simulink model "AMR_main_23b"  (R2024a)
settings: configuration reference "Configuration" (kept outside this file)
model workspace (MAT data in the model file):
  RTK_health_condition = 30
  mdlWSDbList : string (value not decoded)
undefined symbols (not defined in the file or in its folder): Down, Pull
libraries: speedgoatlib_IO60X_IO69X x17, tramontina_database_nvidialib x11, tramontina_database_curtislib x7, tramontina_database_xsenslib x4, tramontina_database_moboticlib x4, speedgoatlib_IO691 x3, canmsglib x2, slrealtimeseriallib x2, etargetslib x1, tramontina_database_sick_modbuslib x1
(part 2 of 2)

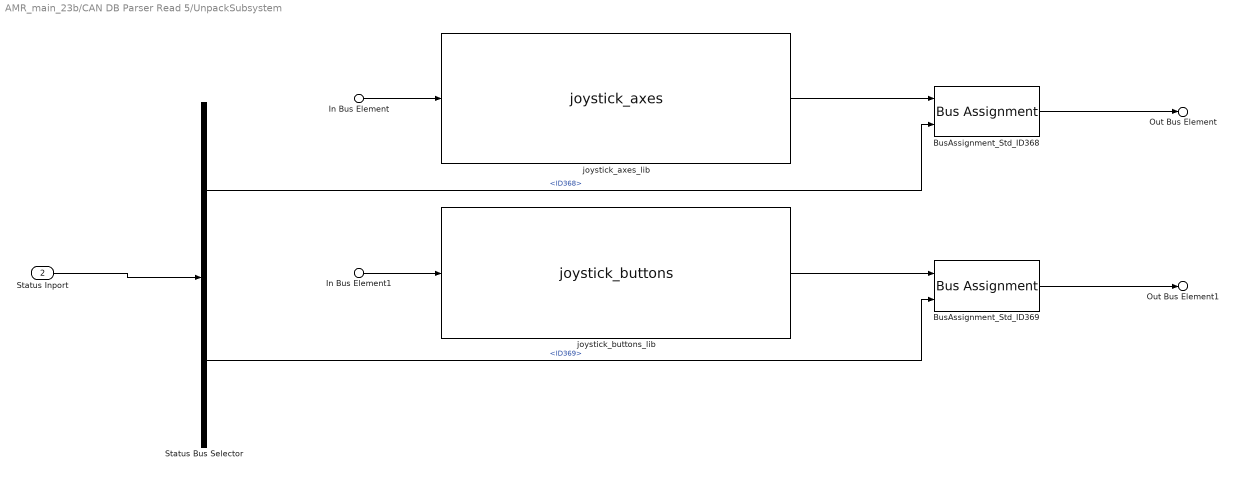
== system AMR_main_23b/CAN DB Parser Read 5/UnpackSubsystem ==
  In Bus Element : Inport  PortName=Unpack_In  Element=Std.ID368
  In Bus Element1 : Inport  PortName=Unpack_In  Element=Std.ID369
  Status Inport : Inport  Port=2
  BusAssignment_Std_ID368 : BusAssignment  AssignedSignals=MessageStatus.Status
  BusAssignment_Std_ID369 : BusAssignment  AssignedSignals=MessageStatus.Status
  Status Bus Selector : BusSelector  OutputSignals=Std.ID368,Std.ID369
  joystick_axes_lib : tramontina_database_nvidialib/CAN unpack/joystick_axes  SystemSampleTime=-1  VariantActivationTime=update diagram  AllowFlexibleInterface=on  Latency=0  AutoFrameSizeCalculation=off
  joystick_buttons_lib : tramontina_database_nvidialib/CAN unpack/joystick_buttons  SystemSampleTime=-1  VariantActivationTime=update diagram  AllowFlexibleInterface=on  Latency=0  AutoFrameSizeCalculation=off
  Out Bus Element : Outport  PortName=Unpack_Out  Element=ID368_joystick_axes
  Out Bus Element1 : Outport  PortName=Unpack_Out  Element=ID369_joystick_buttons
  wires:
  In Bus Element/1 -> joystick_axes_lib/1
  joystick_axes_lib/1 -> BusAssignment_Std_ID368/1
  BusAssignment_Std_ID368/1 -> Out Bus Element/1
  In Bus Element1/1 -> joystick_buttons_lib/1
  joystick_buttons_lib/1 -> BusAssignment_Std_ID369/1
  BusAssignment_Std_ID369/1 -> Out Bus Element1/1
  Status Inport/1 -> Status Bus Selector/1
  Status Bus Selector/1 -> BusAssignment_Std_ID368/2  "<ID368>"
  Status Bus Selector/2 -> BusAssignment_Std_ID369/2  "<ID369>"

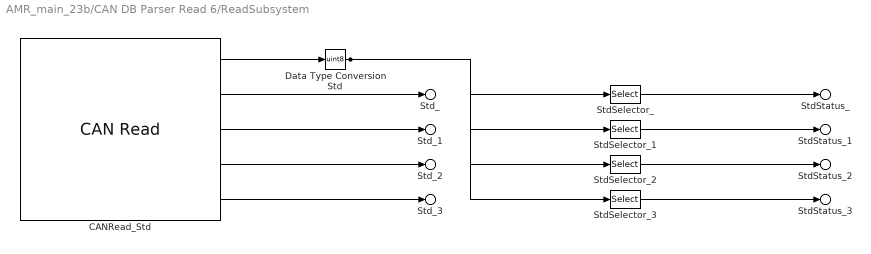
== system AMR_main_23b/CAN DB Parser Read 6/ReadSubsystem ==
  CANRead_Std : speedgoatlib_IO60X_IO69X/CAN/CAN Read   moduleType=IO691  id=1  channel=1  canType=CAN (HS)  messageType=CAN (HS)  useBusOut=on  HasMulRead=Specify by IDs  MsgIDlist="[370  371  372  373]"  isEFF=off  LabelInHex=off  enableInput=off  initValues=[691 1 0.005 0 1 1 0 1 2 0 4 370 371 372 373]  ts=5e-3
  Data Type ConversionStd : DataTypeConversion  OutDataTypeStr=uint8  SaturateOnIntegerOverflow=off  RndMeth=Floor
  StdSelector_ : Selector  IndexOptions=Index vector (dialog)  Indices=1  OutputSizes=1
  StdSelector_1 : Selector  IndexOptions=Index vector (dialog)  Indices=2  OutputSizes=1
  StdSelector_2 : Selector  IndexOptions=Index vector (dialog)  Indices=3  OutputSizes=1
  StdSelector_3 : Selector  IndexOptions=Index vector (dialog)  Indices=4  OutputSizes=1
  Std_ : Outport  PortName=Raw_Rx  Element=Std.ID370
  Std_1 : Outport  PortName=Raw_Rx  Element=Std.ID371
  Std_2 : Outport  PortName=Raw_Rx  Element=Std.ID372
  Std_3 : Outport  PortName=Raw_Rx  Element=Std.ID373
  StdStatus_ : Outport  Port=2  PortName=Status_Rx  Element=Std.ID370
  StdStatus_1 : Outport  Port=2  PortName=Status_Rx  Element=Std.ID371
  StdStatus_2 : Outport  Port=2  PortName=Status_Rx  Element=Std.ID372
  StdStatus_3 : Outport  Port=2  PortName=Status_Rx  Element=Std.ID373
  wires:
  CANRead_Std/1 -> Data Type ConversionStd/1
  CANRead_Std/2 -> Std_/1
  CANRead_Std/3 -> Std_1/1
  CANRead_Std/4 -> Std_2/1
  CANRead_Std/5 -> Std_3/1
  Data Type ConversionStd/1 -> StdSelector_/1, StdSelector_1/1, StdSelector_2/1, StdSelector_3/1
  StdSelector_/1 -> StdStatus_/1
  StdSelector_1/1 -> StdStatus_1/1
  StdSelector_2/1 -> StdStatus_2/1
  StdSelector_3/1 -> StdStatus_3/1

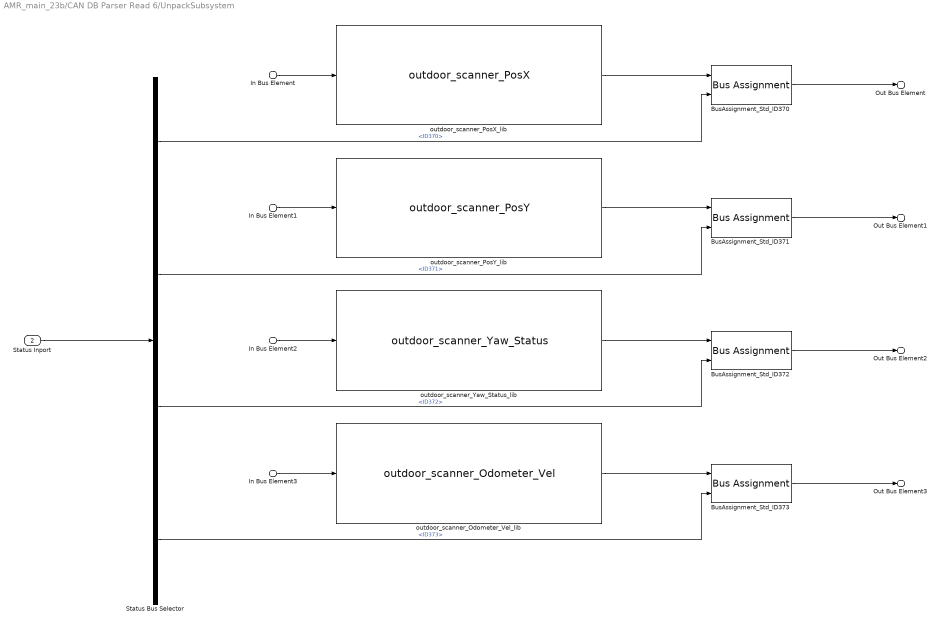
== system AMR_main_23b/CAN DB Parser Read 6/UnpackSubsystem ==
  In Bus Element : Inport  PortName=Unpack_In  Element=Std.ID370
  In Bus Element1 : Inport  PortName=Unpack_In  Element=Std.ID371
  In Bus Element2 : Inport  PortName=Unpack_In  Element=Std.ID372
  In Bus Element3 : Inport  PortName=Unpack_In  Element=Std.ID373
  Status Inport : Inport  Port=2
  BusAssignment_Std_ID{370..373} (4 alike) : BusAssignment  AssignedSignals=MessageStatus.Status
  Status Bus Selector : BusSelector  OutputSignals=Std.ID370,Std.ID371,Std.ID372,Std.ID373
  outdoor_scanner_Odometer_Vel_lib : tramontina_database_nvidialib/CAN unpack/outdoor_scanner_Odometer_Vel  SystemSampleTime=-1  VariantActivationTime=update diagram  AllowFlexibleInterface=on  Latency=0  AutoFrameSizeCalculation=off
  outdoor_scanner_PosX_lib : tramontina_database_nvidialib/CAN unpack/outdoor_scanner_PosX  SystemSampleTime=-1  VariantActivationTime=update diagram  AllowFlexibleInterface=on  Latency=0  AutoFrameSizeCalculation=off
  outdoor_scanner_PosY_lib : tramontina_database_nvidialib/CAN unpack/outdoor_scanner_PosY  SystemSampleTime=-1  VariantActivationTime=update diagram  AllowFlexibleInterface=on  Latency=0  AutoFrameSizeCalculation=off
  outdoor_scanner_Yaw_Status_lib : tramontina_database_nvidialib/CAN unpack/outdoor_scanner_Yaw_Status  SystemSampleTime=-1  VariantActivationTime=update diagram  AllowFlexibleInterface=on  Latency=0  AutoFrameSizeCalculation=off
  Out Bus Element : Outport  PortName=Unpack_Out  Element=ID370_outdoor_scanner_PosX
  Out Bus Element1 : Outport  PortName=Unpack_Out  Element=ID371_outdoor_scanner_PosY
  Out Bus Element2 : Outport  PortName=Unpack_Out  Element=ID372_outdoor_scanner_Yaw_Status
  Out Bus Element3 : Outport  PortName=Unpack_Out  Element=ID373_outdoor_scanner_Odometer_Vel
  wires:
  In Bus Element/1 -> outdoor_scanner_PosX_lib/1
  outdoor_scanner_PosX_lib/1 -> BusAssignment_Std_ID370/1
  BusAssignment_Std_ID370/1 -> Out Bus Element/1
  In Bus Element1/1 -> outdoor_scanner_PosY_lib/1
  outdoor_scanner_PosY_lib/1 -> BusAssignment_Std_ID371/1
  BusAssignment_Std_ID371/1 -> Out Bus Element1/1
  In Bus Element2/1 -> outdoor_scanner_Yaw_Status_lib/1
  outdoor_scanner_Yaw_Status_lib/1 -> BusAssignment_Std_ID372/1
  BusAssignment_Std_ID372/1 -> Out Bus Element2/1
  In Bus Element3/1 -> outdoor_scanner_Odometer_Vel_lib/1
  outdoor_scanner_Odometer_Vel_lib/1 -> BusAssignment_Std_ID373/1
  BusAssignment_Std_ID373/1 -> Out Bus Element3/1
  Status Inport/1 -> Status Bus Selector/1
  Status Bus Selector/1 -> BusAssignment_Std_ID370/2  "<ID370>"
  Status Bus Selector/2 -> BusAssignment_Std_ID371/2  "<ID371>"
  Status Bus Selector/3 -> BusAssignment_Std_ID372/2  "<ID372>"
  Status Bus Selector/4 -> BusAssignment_Std_ID373/2  "<ID373>"

== system AMR_main_23b/CAN DB Parser Read 7/ReadSubsystem ==
  CANRead_Std : speedgoatlib_IO60X_IO69X/CAN/CAN Read   moduleType=IO691  id=1  channel=1  canType=CAN (HS)  messageType=CAN (HS)  useBusOut=on  HasMulRead=Specify by IDs  MsgIDlist=[1459]  isEFF=off  LabelInHex=off  enableInput=off  initValues=[691 1 0.005 0 1 1 0 1 2 0 1 1459]  ts=5e-3
  Data Type ConversionStd : DataTypeConversion  OutDataTypeStr=uint8  SaturateOnIntegerOverflow=off  RndMeth=Floor
  StdSelector_ : Selector  IndexOptions=Index vector (dialog)  Indices=1  OutputSizes=1
  Std_ : Outport  PortName=Raw_Rx  Element=Std.ID1459
  StdStatus_ : Outport  Port=2  PortName=Status_Rx  Element=Std.ID1459
  wires:
  CANRead_Std/1 -> Data Type ConversionStd/1
  CANRead_Std/2 -> Std_/1
  Data Type ConversionStd/1 -> StdSelector_/1
  StdSelector_/1 -> StdStatus_/1

== system AMR_main_23b/CAN DB Parser Read 7/UnpackSubsystem ==
  In Bus Element : Inport  PortName=Unpack_In  Element=Std.ID1459
  Status Inport : Inport  Port=2
  BusAssignment_Std_ID1459 : BusAssignment  AssignedSignals=MessageStatus.Status
  Status Bus Selector : BusSelector  OutputSignals=Std.ID1459
  feedback_word_lib : tramontina_database_moboticlib/CAN unpack/feedback_word  SystemSampleTime=-1  VariantActivationTime=update diagram  AllowFlexibleInterface=on  Latency=0  AutoFrameSizeCalculation=off
  Out Bus Element : Outport  PortName=Unpack_Out  Element=ID1459_feedback_word
  wires:
  In Bus Element/1 -> feedback_word_lib/1
  feedback_word_lib/1 -> BusAssignment_Std_ID1459/1
  BusAssignment_Std_ID1459/1 -> Out Bus Element/1
  Status Inport/1 -> Status Bus Selector/1
  Status Bus Selector/1 -> BusAssignment_Std_ID1459/2  "<ID1459>"

== system AMR_main_23b/CAN DB Parser Write /BusMapping ==
  AMR_auto_mode : Inport  PortName=InBus  Element=AMR_auto_mode
  AMR_idle_mode : Inport  PortName=InBus  Element=AMR_idle_mode
  AMR_manual_mode : Inport  PortName=InBus  Element=AMR_manual_mode
  ID344_AMR_OperationMode_feedback.OperationMode_auto : Outport  PortName=OutBus  Element=ID344_AMR_OperationMode_feedback.OperationMode_auto
  ID344_AMR_OperationMode_feedback.OperationMode_idle : Outport  PortName=OutBus  Element=ID344_AMR_OperationMode_feedback.OperationMode_idle
  ID344_AMR_OperationMode_feedback.OperationMode_manual : Outport  PortName=OutBus  Element=ID344_AMR_OperationMode_feedback.OperationMode_manual
  wires:
  AMR_auto_mode/1 -> ID344_AMR_OperationMode_feedback.OperationMode_auto/1
  AMR_idle_mode/1 -> ID344_AMR_OperationMode_feedback.OperationMode_idle/1
  AMR_manual_mode/1 -> ID344_AMR_OperationMode_feedback.OperationMode_manual/1

== system AMR_main_23b/CAN DB Parser Write /Convert2BusArray ==
  In1 : Inport  PortName=InBus  Element=ID344_AMR_OperationMode_feedback
  BusArray : Concatenate  NumInputs=1
  BusArrayOut : Outport
  wires:
  In1/1 -> BusArray/1
  BusArray/1 -> BusArrayOut/1

== system AMR_main_23b/CAN DB Parser Write /PackSubsystem ==
  In Bus Element : Inport  PortName=PackIn  Element=ID344_AMR_OperationMode_feedback
  AMR_OperationMode_feedback_lib : tramontina_database_nvidialib/CAN pack/AMR_OperationMode_feedback  SystemSampleTime=-1  VariantActivationTime=update diagram  AllowFlexibleInterface=on  Latency=0  AutoFrameSizeCalculation=off
  In Bus Element1 : Outport  PortName=PackOut  Element=ID344_AMR_OperationMode_feedback
  wires:
  In Bus Element/1 -> AMR_OperationMode_feedback_lib/1
  AMR_OperationMode_feedback_lib/1 -> In Bus Element1/1

== system AMR_main_23b/CAN DB Parser Write 1/Convert2BusArray ==
  In1 : Inport  PortName=InBus  Element=ID290_AMR_vehicle_speed
  BusArray : Concatenate  NumInputs=1
  BusArrayOut : Outport
  wires:
  In1/1 -> BusArray/1
  BusArray/1 -> BusArrayOut/1

== system AMR_main_23b/CAN DB Parser Write 1/InputSubsystem ==
  In1_1 : Inport
  In1_2 : Inport  Port=2
  ID290_AMR_vehicle_speed.speed_m_per_min : Outport  PortName=OutBus  Element=ID290_AMR_vehicle_speed.speed_m_per_min
  ID290_AMR_vehicle_speed.speed_m_per_s : Outport  PortName=OutBus  Element=ID290_AMR_vehicle_speed.speed_m_per_s
  wires:
  In1_1/1 -> ID290_AMR_vehicle_speed.speed_m_per_min/1
  In1_2/1 -> ID290_AMR_vehicle_speed.speed_m_per_s/1

== system AMR_main_23b/CAN DB Parser Write 1/PackSubsystem ==
  In Bus Element : Inport  PortName=PackIn  Element=ID290_AMR_vehicle_speed
  AMR_vehicle_speed_lib : tramontina_database_nvidialib/CAN pack/AMR_vehicle_speed  SystemSampleTime=-1  VariantActivationTime=update diagram  AllowFlexibleInterface=on  Latency=0  AutoFrameSizeCalculation=off
  In Bus Element1 : Outport  PortName=PackOut  Element=ID290_AMR_vehicle_speed
  wires:
  In Bus Element/1 -> AMR_vehicle_speed_lib/1
  AMR_vehicle_speed_lib/1 -> In Bus Element1/1

== system AMR_main_23b/CAN DB Parser Write 2/BusMapping ==
  signal1 : Inport  PortName=InBus  Element=signal1
  signal2 : Inport  PortName=InBus  Element=signal2
  ID550_curtis_input_message_left.rpm_set_left : Outport  PortName=OutBus  Element=ID550_curtis_input_message_left.rpm_set_left
  ID551_curtis_input_message_right.rpm_set_right : Outport  PortName=OutBus  Element=ID551_curtis_input_message_right.rpm_set_right
  wires:
  signal1/1 -> ID550_curtis_input_message_left.rpm_set_left/1
  signal2/1 -> ID551_curtis_input_message_right.rpm_set_right/1

== system AMR_main_23b/CAN DB Parser Write 2/Convert2BusArray ==
  In1 : Inport  PortName=InBus  Element=ID550_curtis_input_message_left
  In2 : Inport  PortName=InBus  Element=ID551_curtis_input_message_right
  BusArray : Concatenate
  BusArrayOut : Outport
  wires:
  In1/1 -> BusArray/1
  In2/1 -> BusArray/2
  BusArray/1 -> BusArrayOut/1

== system AMR_main_23b/CAN DB Parser Write 2/PackSubsystem ==
  In Bus Element : Inport  PortName=PackIn  Element=ID550_curtis_input_message_left
  In Bus Element2 : Inport  PortName=PackIn  Element=ID551_curtis_input_message_right
  curtis_input_message_left_lib : tramontina_database_curtislib/CAN pack/curtis_input_message_left  SystemSampleTime=-1  VariantActivationTime=update diagram  AllowFlexibleInterface=on  Latency=0  AutoFrameSizeCalculation=off
  curtis_input_message_right_lib : tramontina_database_curtislib/CAN pack/curtis_input_message_right  SystemSampleTime=-1  VariantActivationTime=update diagram  AllowFlexibleInterface=on  Latency=0  AutoFrameSizeCalculation=off
  In Bus Element1 : Outport  PortName=PackOut  Element=ID550_curtis_input_message_left
  In Bus Element3 : Outport  PortName=PackOut  Element=ID551_curtis_input_message_right
  wires:
  In Bus Element/1 -> curtis_input_message_left_lib/1
  curtis_input_message_left_lib/1 -> In Bus Element1/1
  In Bus Element2/1 -> curtis_input_message_right_lib/1
  curtis_input_message_right_lib/1 -> In Bus Element3/1

== system AMR_main_23b/CAN DB Parser Write 3/Convert2BusArray ==
  In1 : Inport  PortName=InBus  Element=ID0_curtis_input_operational
  BusArray : Concatenate  NumInputs=1
  BusArrayOut : Outport
  wires:
  In1/1 -> BusArray/1
  BusArray/1 -> BusArrayOut/1

== system AMR_main_23b/CAN DB Parser Write 3/InputSubsystem ==
  In1_1 : Inport
  ID0_curtis_input_operational.pre_operational : Outport  PortName=OutBus  Element=ID0_curtis_input_operational.pre_operational
  wires:
  In1_1/1 -> ID0_curtis_input_operational.pre_operational/1

== system AMR_main_23b/CAN DB Parser Write 3/PackSubsystem ==
  In Bus Element : Inport  PortName=PackIn  Element=ID0_curtis_input_operational
  curtis_input_operational_lib : tramontina_database_curtislib/CAN pack/curtis_input_operational  SystemSampleTime=-1  VariantActivationTime=update diagram  AllowFlexibleInterface=on  Latency=0  AutoFrameSizeCalculation=off
  In Bus Element1 : Outport  PortName=PackOut  Element=ID0_curtis_input_operational
  wires:
  In Bus Element/1 -> curtis_input_operational_lib/1
  curtis_input_operational_lib/1 -> In Bus Element1/1

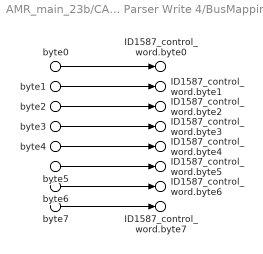
== system AMR_main_23b/CAN DB Parser Write 4/BusMapping ==
  byte0 : Inport  PortName=InBus  Element=byte0
  byte1 : Inport  PortName=InBus  Element=byte1
  byte2 : Inport  PortName=InBus  Element=byte2
  byte3 : Inport  PortName=InBus  Element=byte3
  byte4 : Inport  PortName=InBus  Element=byte4
  byte5 : Inport  PortName=InBus  Element=byte5
  byte6 : Inport  PortName=InBus  Element=byte6
  byte7 : Inport  PortName=InBus  Element=byte7
  ID1587_control_word.byte0 : Outport  PortName=OutBus  Element=ID1587_control_word.byte0
  ID1587_control_word.byte1 : Outport  PortName=OutBus  Element=ID1587_control_word.byte1
  ID1587_control_word.byte2 : Outport  PortName=OutBus  Element=ID1587_control_word.byte2
  ID1587_control_word.byte3 : Outport  PortName=OutBus  Element=ID1587_control_word.byte3
  ID1587_control_word.byte4 : Outport  PortName=OutBus  Element=ID1587_control_word.byte4
  ID1587_control_word.byte5 : Outport  PortName=OutBus  Element=ID1587_control_word.byte5
  ID1587_control_word.byte6 : Outport  PortName=OutBus  Element=ID1587_control_word.byte6
  ID1587_control_word.byte7 : Outport  PortName=OutBus  Element=ID1587_control_word.byte7
  wires:
  byte0/1 -> ID1587_control_word.byte0/1
  byte1/1 -> ID1587_control_word.byte1/1
  byte2/1 -> ID1587_control_word.byte2/1
  byte3/1 -> ID1587_control_word.byte3/1
  byte4/1 -> ID1587_control_word.byte4/1
  byte5/1 -> ID1587_control_word.byte5/1
  byte6/1 -> ID1587_control_word.byte6/1
  byte7/1 -> ID1587_control_word.byte7/1

== system AMR_main_23b/CAN DB Parser Write 4/Convert2BusArray ==
  In1 : Inport  PortName=InBus  Element=ID1587_control_word
  BusArray : Concatenate  NumInputs=1
  BusArrayOut : Outport
  wires:
  In1/1 -> BusArray/1
  BusArray/1 -> BusArrayOut/1

== system AMR_main_23b/CAN DB Parser Write 4/PackSubsystem ==
  In Bus Element : Inport  PortName=PackIn  Element=ID1587_control_word
  control_word_lib : tramontina_database_moboticlib/CAN pack/control_word  SystemSampleTime=-1  VariantActivationTime=update diagram  AllowFlexibleInterface=on  Latency=0  AutoFrameSizeCalculation=off
  In Bus Element1 : Outport  PortName=PackOut  Element=ID1587_control_word
  wires:
  In Bus Element/1 -> control_word_lib/1
  control_word_lib/1 -> In Bus Element1/1

== system AMR_main_23b/CAN DB Parser Write 5/Convert2BusArray ==
  In1 : Inport  PortName=InBus  Element=ID289_mobotic_error_flag
  BusArray : Concatenate  NumInputs=1
  BusArrayOut : Outport
  wires:
  In1/1 -> BusArray/1
  BusArray/1 -> BusArrayOut/1

== system AMR_main_23b/CAN DB Parser Write 5/InputSubsystem ==
  In1_1 : Inport
  ID289_mobotic_error_flag.steering_unit_error : Outport  PortName=OutBus  Element=ID289_mobotic_error_flag.steering_unit_error
  wires:
  In1_1/1 -> ID289_mobotic_error_flag.steering_unit_error/1

== system AMR_main_23b/CAN DB Parser Write 5/PackSubsystem ==
  In Bus Element : Inport  PortName=PackIn  Element=ID289_mobotic_error_flag
  mobotic_error_flag_lib : tramontina_database_nvidialib/CAN pack/mobotic_error_flag  SystemSampleTime=-1  VariantActivationTime=update diagram  AllowFlexibleInterface=on  Latency=0  AutoFrameSizeCalculation=off
  In Bus Element1 : Outport  PortName=PackOut  Element=ID289_mobotic_error_flag
  wires:
  In Bus Element/1 -> mobotic_error_flag_lib/1
  mobotic_error_flag_lib/1 -> In Bus Element1/1

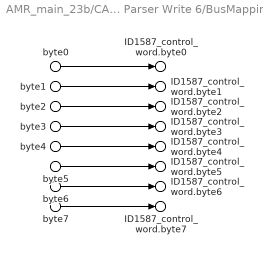
== system AMR_main_23b/CAN DB Parser Write 6/BusMapping ==
  byte0 : Inport  PortName=InBus  Element=byte0
  byte1 : Inport  PortName=InBus  Element=byte1
  byte2 : Inport  PortName=InBus  Element=byte2
  byte3 : Inport  PortName=InBus  Element=byte3
  byte4 : Inport  PortName=InBus  Element=byte4
  byte5 : Inport  PortName=InBus  Element=byte5
  byte6 : Inport  PortName=InBus  Element=byte6
  byte7 : Inport  PortName=InBus  Element=byte7
  ID1587_control_word.byte0 : Outport  PortName=OutBus  Element=ID1587_control_word.byte0
  ID1587_control_word.byte1 : Outport  PortName=OutBus  Element=ID1587_control_word.byte1
  ID1587_control_word.byte2 : Outport  PortName=OutBus  Element=ID1587_control_word.byte2
  ID1587_control_word.byte3 : Outport  PortName=OutBus  Element=ID1587_control_word.byte3
  ID1587_control_word.byte4 : Outport  PortName=OutBus  Element=ID1587_control_word.byte4
  ID1587_control_word.byte5 : Outport  PortName=OutBus  Element=ID1587_control_word.byte5
  ID1587_control_word.byte6 : Outport  PortName=OutBus  Element=ID1587_control_word.byte6
  ID1587_control_word.byte7 : Outport  PortName=OutBus  Element=ID1587_control_word.byte7
  wires:
  byte0/1 -> ID1587_control_word.byte0/1
  byte1/1 -> ID1587_control_word.byte1/1
  byte2/1 -> ID1587_control_word.byte2/1
  byte3/1 -> ID1587_control_word.byte3/1
  byte4/1 -> ID1587_control_word.byte4/1
  byte5/1 -> ID1587_control_word.byte5/1
  byte6/1 -> ID1587_control_word.byte6/1
  byte7/1 -> ID1587_control_word.byte7/1

== system AMR_main_23b/CAN DB Parser Write 6/Convert2BusArray ==
  In1 : Inport  PortName=InBus  Element=ID1587_control_word
  BusArray : Concatenate  NumInputs=1
  BusArrayOut : Outport
  wires:
  In1/1 -> BusArray/1
  BusArray/1 -> BusArrayOut/1

== system AMR_main_23b/CAN DB Parser Write 6/PackSubsystem ==
  In Bus Element : Inport  PortName=PackIn  Element=ID1587_control_word
  control_word_lib : tramontina_database_moboticlib/CAN pack/control_word  SystemSampleTime=-1  VariantActivationTime=update diagram  AllowFlexibleInterface=on  Latency=0  AutoFrameSizeCalculation=off
  In Bus Element1 : Outport  PortName=PackOut  Element=ID1587_control_word
  wires:
  In Bus Element/1 -> control_word_lib/1
  control_word_lib/1 -> In Bus Element1/1

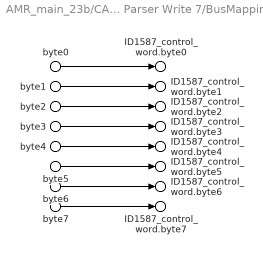
== system AMR_main_23b/CAN DB Parser Write 7/BusMapping ==
  byte0 : Inport  PortName=InBus  Element=byte0
  byte1 : Inport  PortName=InBus  Element=byte1
  byte2 : Inport  PortName=InBus  Element=byte2
  byte3 : Inport  PortName=InBus  Element=byte3
  byte4 : Inport  PortName=InBus  Element=byte4
  byte5 : Inport  PortName=InBus  Element=byte5
  byte6 : Inport  PortName=InBus  Element=byte6
  byte7 : Inport  PortName=InBus  Element=byte7
  ID1587_control_word.byte0 : Outport  PortName=OutBus  Element=ID1587_control_word.byte0
  ID1587_control_word.byte1 : Outport  PortName=OutBus  Element=ID1587_control_word.byte1
  ID1587_control_word.byte2 : Outport  PortName=OutBus  Element=ID1587_control_word.byte2
  ID1587_control_word.byte3 : Outport  PortName=OutBus  Element=ID1587_control_word.byte3
  ID1587_control_word.byte4 : Outport  PortName=OutBus  Element=ID1587_control_word.byte4
  ID1587_control_word.byte5 : Outport  PortName=OutBus  Element=ID1587_control_word.byte5
  ID1587_control_word.byte6 : Outport  PortName=OutBus  Element=ID1587_control_word.byte6
  ID1587_control_word.byte7 : Outport  PortName=OutBus  Element=ID1587_control_word.byte7
  wires:
  byte0/1 -> ID1587_control_word.byte0/1
  byte1/1 -> ID1587_control_word.byte1/1
  byte2/1 -> ID1587_control_word.byte2/1
  byte3/1 -> ID1587_control_word.byte3/1
  byte4/1 -> ID1587_control_word.byte4/1
  byte5/1 -> ID1587_control_word.byte5/1
  byte6/1 -> ID1587_control_word.byte6/1
  byte7/1 -> ID1587_control_word.byte7/1

== system AMR_main_23b/CAN DB Parser Write 7/Convert2BusArray ==
  In1 : Inport  PortName=InBus  Element=ID1587_control_word
  BusArray : Concatenate  NumInputs=1
  BusArrayOut : Outport
  wires:
  In1/1 -> BusArray/1
  BusArray/1 -> BusArrayOut/1

== system AMR_main_23b/CAN DB Parser Write 7/PackSubsystem ==
  In Bus Element : Inport  PortName=PackIn  Element=ID1587_control_word
  control_word_lib : tramontina_database_moboticlib/CAN pack/control_word  SystemSampleTime=-1  VariantActivationTime=update diagram  AllowFlexibleInterface=on  Latency=0  AutoFrameSizeCalculation=off
  In Bus Element1 : Outport  PortName=PackOut  Element=ID1587_control_word
  wires:
  In Bus Element/1 -> control_word_lib/1
  control_word_lib/1 -> In Bus Element1/1
